simulink model "Model_plane9Old_vers"  (R2021a)
settings: Solver=FixedStepAuto  StartTime=0  StopTime=3000  FixedStep=0.1  RelTol=1e-3
model workspace (MAT data in the model file):
  Alfa = [-2 4 10 16]
  Alfa_RUD = 0.7
  Alfa_table = [-4 0 5 10 20]
  Alfa_y = [-4 6 8 9 10 12 14]
  Cxa_table = [0.03434  0.0358  0.04274; 0.02598  0.0252  0.0262; 0.04151  0.0505  0.0883; 0.122  0.1649  0.2341; 0.502  0.538  0.666]
  Cy_DB = [0.01242 0.01286 0.01457]
  Cy_fi = [0.00623 0.00643 0.00626]
  Cya = [-0.276  -0.33  -0.39; 0.859  0.991  0.82; 1.085  1.211  1.1; 1.2  1.275  1.031; 1.296  1.29  1.018; 1.45  1.178  1.043; 1.461  1.163  1.081]
  Del_B = -5
  H = [339 3256 4060 8000 12000]
  H0 = 5000
  H_table = [0 2000 4000 6000 8000 10000]
  L0 = 0
  M_C = [0.4 0.6 0.82]
  M_mz = [0.2 0.4 0.6 0.8]
  M_mz2 = [0.4 0.7 0.85]
  M_table = [0.4 0.7 0.82]
  M_y = [0.4 0.7 0.82]
  P = [50000 40000 32000 25600 20480]
  Skr = 131
  Vx0 = 160
  Vy0 = 0
  a_table = [340.3 339.5 338.8 338 337.2 336.4]
  ba = 3.466
  fi = 0
  fi_P = 2
  g = 9.81
  lz = 4500000
  mla = 60000
  mz_DB = [-0.035 -0.0358 -0.037 -0.0377]
  mz_alfa = [-0.0282 -0.0282 -0.0289 -0.0404]
  mz_alfa2 = [-8.163  -8.762  -9.714; -8.163  -8.762  -9.583; -7.975  -7.991  -7.868; -6.514  -6.413  -6.732]
  mz_fi = [-0.0695 -0.0714 -0.0739 -0.0832]
  mz_omz = [-23.768  -25.3  -28.284; -23.768  -25.3  -27.903; -23.222  -22.6  -23.32; -18.967  -18.52  -19.601]
  n_dvig = 2
  out = Simulink.SimulationOutput
  out.Data.tout = [0 1.67688873362e-06 9.33181354111e-06 4.76064375786e-05 0.000238979557766 0.0011958451587 0.00598017316339 0.0291858115735 0.107609227908 0.294605508218 0.534390352194 0.619831316604 ... (6422 elements, 6422x1)]
  out.Metadata = Simulink.SimulationMetadata
  out.Metadata.ModelInfo.ModelName = 'Model_plane2'
  out.Metadata.ModelInfo.ModelVersion = '1.11'
  out.Metadata.ModelInfo.ModelFilePath = 'C:\Users\Анастасия\Универ\Mathlab\Модель самолёта\Model_plane2.slx'
  out.Metadata.ModelInfo.UserID = 'Анастасия'
  out.Metadata.ModelInfo.MachineName = 'DESKTOP-OE36224'
  out.Metadata.ModelInfo.Platform = 'PCWIN64'
  out.Metadata.ModelInfo.ModelStructuralChecksum = [329193822; 1830100004; 2373400892; 4162968501]
  out.Metadata.ModelInfo.SimulationMode = 'normal'
  out.Metadata.ModelInfo.StartTime = 0
  out.Metadata.ModelInfo.StopTime = 100
  out.Metadata.ModelInfo.SolverInfo.Type = 'Variable-Step'
  out.Metadata.ModelInfo.SolverInfo.Solver = 'ode45'
  out.Metadata.ModelInfo.SolverInfo.MaxStepSize = 2
  out.Metadata.ModelInfo.SimulinkVersion.Name = 'Simulink'
  out.Metadata.ModelInfo.SimulinkVersion.Version = '24.1'
  out.Metadata.ModelInfo.SimulinkVersion.Release = '(R2024a)'
  out.Metadata.ModelInfo.SimulinkVersion.Date = '19-Nov-2023'
  out.Metadata.ModelInfo.LoggingInfo.LoggingToFile = 'off'
  out.Metadata.TimingInfo.WallClockTimestampStart = '2025-02-14 11:01:22'
  out.Metadata.TimingInfo.WallClockTimestampStop = '2025-02-14 11:01:24'
  out.Metadata.TimingInfo.InitializationElapsedWallTime = 1.1990057
  out.Metadata.TimingInfo.ExecutionElapsedWallTime = 1.0786509
  out.Metadata.TimingInfo.TerminationElapsedWallTime = 0.0112241
  out.Metadata.TimingInfo.TotalElapsedWallTime = 2.2888807
  out.Metadata.TimingInfo.ProfilerData = 'Profiler is not enabled'
  out.Metadata.ExecutionInfo.StopEvent = 'ReachedStopTime'
  out.Metadata.ExecutionInfo.StopEventSource = []
  out.Metadata.ExecutionInfo.StopEventDescription = 'Reached stop time of 100'
  out.Metadata.ExecutionInfo.ErrorDiagnostic = []
  out.Metadata.ExecutionInfo.WarningDiagnostics.Diagnostic = MSLDiagnostic
  out.Metadata.ExecutionInfo.WarningDiagnostics.Diagnostic.identifier = 'Simulink:blocks:DivideByZero'
  out.Metadata.ExecutionInfo.WarningDiagnostics.Diagnostic.message = 'Division by zero in ''<a href="matlab:open_and_hilite_hyperlink (''Model_plane2/Уравнения продольного движения в связанной системе координат/Блок расчёта угла атаки Alfa/Divide'',''error'')">Model_plane2/Уравнения продольного движения в связанной системе координат/Блок расчёта угла атаки Alfa/Divide</a>'''
  out.Metadata.ExecutionInfo.WarningDiagnostics.Diagnostic.paths = {'Model_plane2/Уравнения продольного движения в связанной системе координат/Блок расчёта угла атаки Alfa/Divide'}
  out.Metadata.ExecutionInfo.WarningDiagnostics.Diagnostic.arguments = {'Model_plane2/Уравнения продольного движения в связанной системе координат/Блок расчёта угла атаки Alfa/Divide'}
  out.Metadata.ExecutionInfo.WarningDiagnostics.Diagnostic.stack = struct([])
  out.Metadata.ExecutionInfo.WarningDiagnostics.Diagnostic.actionProp = '22 serialization::archive 19 0 0 0  0 1 0 0 1 1 0 0 0 0 0 1 47 SL_SERVICES:utils:EMBEDDED____ACTION____WRAPPER 2 2 0 0 183 0 109 97 116 108 97 98 58 83 105 109 117 108 105 110 107 46 83 117 112 112 114 101 115 115 101 100 68 105 97 103 110 111 115 116 105 99 40 123 39 77 111 100 101 108 95 112 108 97 110 101 50 47 1059 1088 1072 1074 1085 1077 1085 1080 1103 32 1087 1088 1086 1076 1086 1083 1100 1085 1086 1075 1086 32 1076 1074 1080 1078 1077 1085 1080 1103 32 1074 32 1089 1074 1103 1079 1072 1085 1085 1086 1081 32 1089 1080 1089 1090 1077 1084 1077 32 1082 1086 1086 1088 1076 1080 1085 1072 1090 47 1041 1083 1086 1082 32 1088 1072 1089 1095 1105 1090 1072 32 1091 1075 1083 1072 32 1072 1090 1072 1082 1080 32 65 108 102 97 47 68 105 118 105 100 101 39 125 44 39 83 105 109 117 108 105 110 107 58 98 108 111 99 107 115 58 68 105 118 105 100 101 66 121 90 101 114 111 39 41 59 2 0 0 1 6 0 0 0 0 0  1 0 0 0 0'
  out.Metadata.ExecutionInfo.WarningDiagnostics.Diagnostic.metaDataProp.UI = []
  out.Metadata.ExecutionInfo.WarningDiagnostics.Diagnostic.metaDataProp.STAGE = []
  out.Metadata.ExecutionInfo.WarningDiagnostics.Diagnostic.metaDataProp.CATEGORY = []
  out.Metadata.ExecutionInfo.WarningDiagnostics.Diagnostic.metaDataProp.COMPONENT = []
  out.Metadata.ExecutionInfo.WarningDiagnostics.Diagnostic.metaDataProp.MDL_NAME = []
  out.Metadata.ExecutionInfo.WarningDiagnostics.Diagnostic.metaDataProp.ACTION = '22 serialization::archive 19 0 0 0  0 1 0 0 1 1 0 0 0 0 0 1 47 SL_SERVICES:utils:EMBEDDED____ACTION____WRAPPER 2 2 0 0 183 0 109 97 116 108 97 98 58 83 105 109 117 108 105 110 107 46 83 117 112 112 114 101 115 115 101 100 68 105 97 103 110 111 115 116 105 99 40 123 39 77 111 100 101 108 95 112 108 97 110 101 50 47 1059 1088 1072 1074 1085 1077 1085 1080 1103 32 1087 1088 1086 1076 1086 1083 1100 1085 1086 1075 1086 32 1076 1074 1080 1078 1077 1085 1080 1103 32 1074 32 1089 1074 1103 1079 1072 1085 1085 1086 1081 32 1089 1080 1089 1090 1077 1084 1077 32 1082 1086 1086 1088 1076 1080 1085 1072 1090 47 1041 1083 1086 1082 32 1088 1072 1089 1095 1105 1090 1072 32 1091 1075 1083 1072 32 1072 1090 1072 1082 1080 32 65 108 102 97 47 68 105 118 105 100 101 39 125 44 39 83 105 109 117 108 105 110 107 58 98 108 111 99 107 115 58 68 105 118 105 100 101 66 121 90 101 114 111 39 41 59 2 0 0 1 6 0 0 0 0 0  1 0 0 0 0'
  out.Metadata.ExecutionInfo.WarningDiagnostics.Diagnostic.metaDataProp.DOC = []
  out.Metadata.ExecutionInfo.WarningDiagnostics.Diagnostic.metaDataProp.SUB_CATEGORY = []
  out.Metadata.ExecutionInfo.WarningDiagnostics.Diagnostic.metaDataProp.MSTACK_PRESERVE = []
  out.Metadata.ExecutionInfo.WarningDiagnostics.Diagnostic.metaDataProp.DOUBLE_ARGS = []
  out.Metadata.ExecutionInfo.WarningDiagnostics.Diagnostic.metaDataProp.USER_DATA = []
  out.Metadata.ExecutionInfo.WarningDiagnostics.Diagnostic.priority = 2
  out.Metadata.ExecutionInfo.WarningDiagnostics.SimulationPhase = 'Execution'
  out.Metadata.ExecutionInfo.WarningDiagnostics.SimulationTime = 0
  out.Metadata.AppInfo = struct()
  pitch0 = 0
  q_table = [1.225 1.0065 0.8194 0.6601 0.5258 0.4135]
  wz0 = 0
  xy = [24000 6200]
libraries: simulink x1
settings Model: Creator=Анастасия  LastModifiedBy=Анастасия
settings SolverCC: MaxConsecutiveMinStep=5
settings DebuggingCC: UnconnectedInputMsg=none  UnconnectedOutputMsg=none  UnconnectedLineMsg=none
settings ModelReferenceCC: EnableRefExpFcnMdlSchedulingChecks=off
settings RTWCC: Description=Generic Real-Time Target  GPUComputeCapability=5.0  DLArmComputeVersion=20.02.1

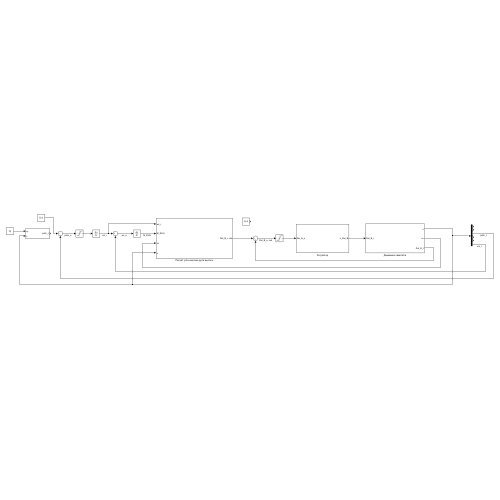
[thumbnail: Simulink's stored preview of the top-level diagram]
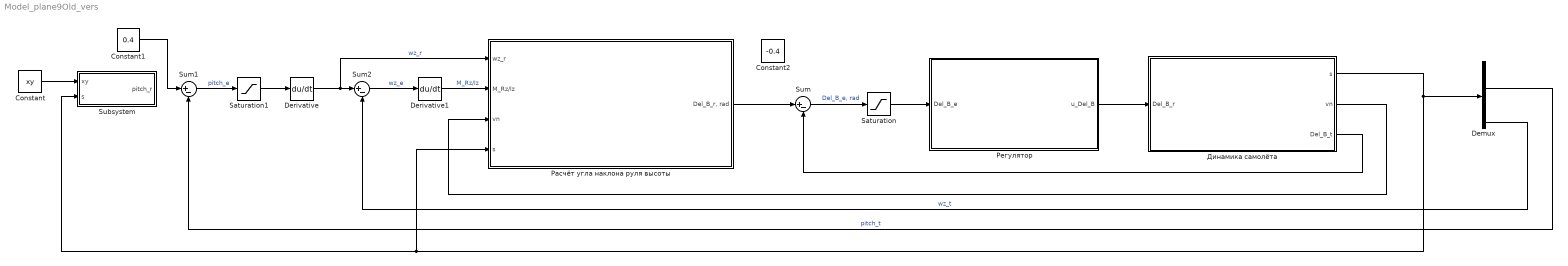
== system Model_plane9Old_vers ==
  Constant : Constant  Value=xy
  Constant1 : Constant  Value=0.4
  Constant2 : Constant  Value=-0.4
  Demux : Demux  Outputs=6
  Derivative : Derivative
  Derivative1 : Derivative
  Saturation : Saturate  UpperLimit=+0.44  LowerLimit=-0.52
  Saturation1 : Saturate  UpperLimit=+80  LowerLimit=-80
  Subsystem : Subsystem
  Sum : Sum  Inputs=|+-
  Sum1 : Sum  Inputs=|+-
  Sum2 : Sum  Inputs=|+-
  Динамика самолёта : Subsystem
  Расчёт угла наклона руля высоты : Subsystem
  Регулятор : Subsystem
  wires:
  Регулятор/1(u_Del_B) -> Динамика самолёта/1(Del_B_r)
  Sum/1 -> Saturation/1  "Del_B_e, rad"
  Динамика самолёта/1(s) -> Subsystem/2(s), Расчёт угла наклона руля высоты/4(s), Demux/1
  Constant/1 -> Subsystem/1(xy)
  Demux/3 -> Sum1/2  "pitch_t"
  Sum1/1 -> Saturation1/1  "pitch_e"
  Saturation1/1 -> Derivative/1
  Derivative/1 -> Расчёт угла наклона руля высоты/1(wz_r), Sum2/1  "wz_r"
  Demux/6 -> Sum2/2  "wz_t"
  Sum2/1 -> Derivative1/1  "wz_e"
  Derivative1/1 -> Расчёт угла наклона руля высоты/2(M_Rz/lz)  "M_Rz/lz"
  Динамика самолёта/2(vn) -> Расчёт угла наклона руля высоты/3(vn)
  Saturation/1 -> Регулятор/1(Del_B_e)
  Динамика самолёта/3(Del_B_t) -> Sum/2
  Расчёт угла наклона руля высоты/1("Del_B_r, rad") -> Sum/1
  Constant1/1 -> Sum1/1

== system Model_plane9Old_vers/Subsystem ==
  xy : Inport
  s : Inport  Port=2
  MATLAB Function : MATLAB Function  TreatAsAtomicUnit=on
  pitch_r : Outport
  wires:
  xy/1 -> MATLAB Function/1(xy)
  s/1 -> MATLAB Function/2(s)
  MATLAB Function/1(pitch) -> pitch_r/1

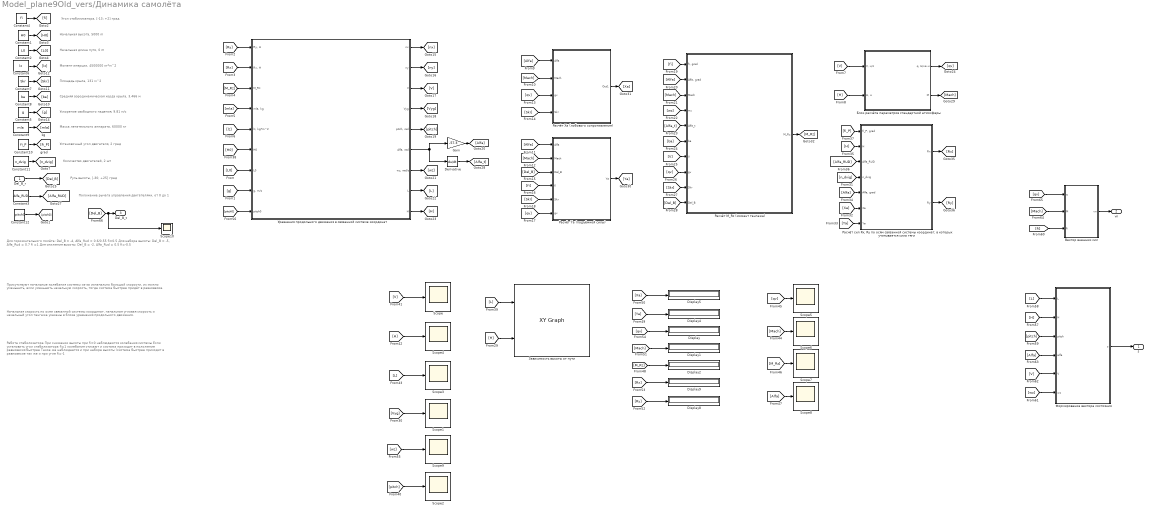
== system Model_plane9Old_vers/Динамика самолёта ==
  note: Руль высоты, [-30; +25] град
  note: Начальная скорость по осям связанной системы координат, начальная угловая скорость и начальный угол тангажа указаны в блоке уравнения продольного движения.
  note: Количество двигателей, 2 шт
  note: Присутствуют начальные колебания системы из-за изначально большой скорости, их можно уменьшить, если уменьшить начальную скорость, тогда система быстрее придёт в равновесие.
  note: Установочный угол двигателя, 2 град
  note: Ускорение свободного падения, 9.81 м/c
  note: Масса летательного аппарата, 60000 кг
  note: Положение рычага управления двигателями, от 0 до 1
  note: Для горизонтального полёта:
      | Del_B = -4, Alfa_Rud = 0.6/0.55 fi=0.5
      | Для набора высоты:
      | Del_B = -5, Alfa_Rud = 0.7 fi =1
      | Для снижения высоты:
      | Del_B = -2, Alfa_Rud = 0.5 fi=-0.5
  note: Начальная длина пути, 0 m
  note: Работа стабилизатора
      | При снижении высоты при fi=0 наблюдаются колебания системы
      | Если установить угол стабилизатора fi=1 колебания стихают и систама приходит в положение равновесия быстрее
      | Такое же наблюдается и при наборе высоты (система быстрее приходит в равновесие так же и при угле fi=-1
  note: Средняя аэродинамическая хорда крыла, 3.466 м
  note: Площадь крыла, 131 м^2
  note: Начальная высота, 5000 m
  note: Момент инерции, 4500000 кг*м^2
  note: Угол стабилизатора, [-13; +2] град
  Del_B_r : Inport
  Constant1 : Constant  Value=H0
  Constant10 : Constant  Value=fi_P
  Constant11 : Constant  Value=n_dvig
  Constant12 : Constant  Value=pitch0
  Constant2 : Constant  Value=L0
  Constant3 : Constant  Value=Alfa_RUD
  Constant4 : Constant  Value=fi
  Constant5 : Constant  Value=g
  Constant6 : Constant  Value=lz
  Constant7 : Constant  Value=Skr
  Constant8 : Constant  Value=ba
  Constant9 : Constant  Value=mla
  Derivative : Derivative
  Display{,1..2,4..5,8..9} (7 alike) : Display
  Gain : Gain  Gain=-57.3
  Scope{,1..10} (11 alike) : Scope
  Блок расчёта параметров стандартной атмосферы : Subsystem
  Вектор внешних сил : Subsystem
  Зависимость высоты от пути : simulink/Sinks/XY Graph  xmin=-1  xmax=1  ymin=-1  ymax=1  st=-1
  Расчёт M_Rz (момент тангажа) : Subsystem
  Расчёт Xa (лобового сопротивления) : Subsystem
  Расчёт Ya (подъёмной силы) : Subsystem
  "Расчёт сил Rx, Ry по осям связанной системы координат, в которых учитывается сила тяги" : Subsystem
  Уравнения продольного движения в связанной системе координат : Subsystem
  Формирование вектора состояния : Subsystem
  s : Outport
  vn : Outport  Port=2
  Del_B_t : Outport  Port=3
  wires:
  [pitch0] -> Уравнения продольного движения в связанной системе координат/9(pitch0)
  Constant12/1 -> [pitch0]
  [wz] -> Scope9/1
  Constant1/1 -> [H0]
  Уравнения продольного движения в связанной системе координат/9(H) -> [H]
  Блок расчёта параметров стандартной атмосферы/1("q, Н/кв.м") -> [qv]
  [M_Rz] -> Display2/1
  [qv] -> Расчёт Ya (подъёмной силы)/6(gv)
  Gain/1 -> [Alfa]
  Расчёт M_Rz (момент тангажа)/1(M_Rz) -> [M_Rz]
  [L0] -> Уравнения продольного движения в связанной системе координат/7(L0)
  [H0] -> Уравнения продольного движения в связанной системе координат/6(H0)
  [qv] -> Display/1
  [Rx] -> Display9/1
  [lz] -> Уравнения продольного движения в связанной системе координат/5("lz, kg*m^2")
  Constant5/1 -> [g]
  [qv] -> Расчёт Xa (лобового сопротивления)/3(gv)
  [pitch] -> Scope2/1
  [Ry] -> Display8/1
  [Vyg] -> Scope1/1
  [Xa] -> Display5/1
  Уравнения продольного движения в связанной системе координат/1(nx) -> [nx]
  Derivative/1 -> [Alfa_t]
  [Mach] -> Display1/1
  [Xa] -> "Расчёт сил Rx, Ry по осям связанной системы координат, в которых учитывается сила тяги"/6(Xa)
  [ba] -> Расчёт M_Rz (момент тангажа)/6(ba)
  [M_Rz] -> Scope7/1
  [Mach] -> Scope6/1
  Constant9/1 -> [mla]
  [H] -> Блок расчёта параметров стандартной атмосферы/2("H, м")
  [Ya] -> Display4/1
  [fi] -> Расчёт M_Rz (момент тангажа)/1("fi, grad")
  [fi_P] -> "Расчёт сил Rx, Ry по осям связанной системы координат, в которых учитывается сила тяги"/1("fi_P, grad")
  [L] -> Scope3/1
  [L] -> Зависимость высоты от пути/1
  [H] -> Scope4/1
  [V] -> Scope/1
  [Ya] -> "Расчёт сил Rx, Ry по осям связанной системы координат, в которых учитывается сила тяги"/7(Ya)
  [V] -> Расчёт M_Rz (момент тангажа)/7(V)
  [Alfa] -> Расчёт M_Rz (момент тангажа)/2("Alfa, grad")
  Уравнения продольного движения в связанной системе координат/5("pitch, rad") -> [pitch]
  [Del_B] -> Расчёт Ya (подъёмной силы)/3(Del_B)
  [Skr] -> Расчёт M_Rz (момент тангажа)/9(Skr)
  [Alfa_RUD] -> "Расчёт сил Rx, Ry по осям связанной системы координат, в которых учитывается сила тяги"/3(Alfa_RUD)
  "Расчёт сил Rx, Ry по осям связанной системы координат, в которых учитывается сила тяги"/1(Rx) -> [Rx]
  [H] -> "Расчёт сил Rx, Ry по осям связанной системы координат, в которых учитывается сила тяги"/2(H)
  [H] -> Зависимость высоты от пути/2
  [fi] -> Расчёт Ya (подъёмной силы)/4(fi)
  Расчёт Xa (лобового сопротивления)/1(Out1) -> [Xa]
  [Del_B] -> Расчёт M_Rz (момент тангажа)/10(Del_B)
  [n_dvig] -> "Расчёт сил Rx, Ry по осям связанной системы координат, в которых учитывается сила тяги"/4(n_dvig)
  [Alfa_t] -> Расчёт M_Rz (момент тангажа)/5(Alfa_t)
  [wz] -> Расчёт M_Rz (момент тангажа)/4(wz)
  Блок расчёта параметров стандартной атмосферы/2(М) -> [Mach]
  Уравнения продольного движения в связанной системе координат/7("wz, rad/s") -> [wz]
  [qv] -> Scope5/1
  [Rx] -> Уравнения продольного движения в связанной системе координат/2("Rx, H")
  Уравнения продольного движения в связанной системе координат/6("Alfa, rad") -> Derivative/1, Gain/1
  "Расчёт сил Rx, Ry по осям связанной системы координат, в которых учитывается сила тяги"/2(Ry) -> [Ry]
  [qv] -> Расчёт M_Rz (момент тангажа)/8(gv)
  [Mach] -> Расчёт Xa (лобового сопротивления)/2(Mach)
  [mla] -> Уравнения продольного движения в связанной системе координат/4("mla, kg")
  [Mach] -> Расчёт Ya (подъёмной силы)/2(Mach)
  Уравнения продольного движения в связанной системе координат/8(L) -> [L]
  [Alfa] -> "Расчёт сил Rx, Ry по осям связанной системы координат, в которых учитывается сила тяги"/5("Alfa, grad")
  [Skr] -> Расчёт Ya (подъёмной силы)/5(Skr)
  [Alfa] -> Расчёт Xa (лобового сопротивления)/1(Alfa)
  Constant10/1 -> [fi_P]
  Constant3/1 -> [Alfa_RUD]
  [M_Rz] -> Уравнения продольного движения в связанной системе координат/3(M_Rz)
  [Mach] -> Расчёт M_Rz (момент тангажа)/3(Mach)
  [V] -> Блок расчёта параметров стандартной атмосферы/1("V, м/с")
  [g] -> Уравнения продольного движения в связанной системе координат/8("g, m/s")
  Уравнения продольного движения в связанной системе координат/2(ny) -> [ny]
  [Alfa] -> Scope8/1
  Уравнения продольного движения в связанной системе координат/4(Vyg) -> [Vyg]
  Расчёт Ya (подъёмной силы)/1(Ya) -> [Ya]
  Уравнения продольного движения в связанной системе координат/3(V) -> [V]
  [Alfa] -> Расчёт Ya (подъёмной силы)/1(Alfa)
  Constant6/1 -> [lz]
  Constant8/1 -> [ba]
  Constant2/1 -> [L0]
  [Ry] -> Уравнения продольного движения в связанной системе координат/1("Ry, H")
  Constant7/1 -> [Skr]
  Constant11/1 -> [n_dvig]
  [Skr] -> Расчёт Xa (лобового сопротивления)/4(Skr)
  Формирование вектора состояния/1(s) -> s/1
  [pitch] -> Формирование вектора состояния/3(pitch)
  [V] -> Формирование вектора состояния/5(V)
  [Alfa] -> Формирование вектора состояния/4(alfa)
  Вектор внешних сил/1(vn) -> vn/1
  [qv] -> Вектор внешних сил/1(q)
  [Mach] -> Вектор внешних сил/2(M)
  Constant4/1 -> [fi]
  [H] -> Формирование вектора состояния/2(H)
  [L] -> Формирование вектора состояния/1(L)
  Del_B_r/1 -> [Del_B]
  [wz] -> Формирование вектора состояния/6(wz)
  [fi] -> Вектор внешних сил/3(fi)
  [Del_B] -> Scope10/1, Del_B_t/1

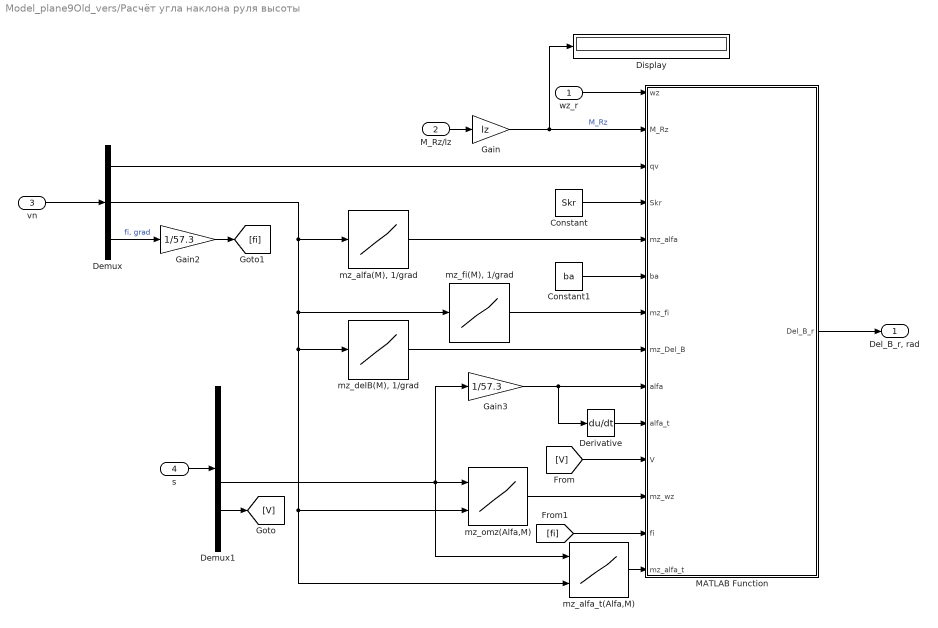
== system Model_plane9Old_vers/Расчёт угла наклона руля высоты ==
  wz_r : Inport
  M_Rz/lz : Inport  Port=2
  vn : Inport  Port=3
  s : Inport  Port=4
  Constant : Constant  Value=Skr
  Constant1 : Constant  Value=ba
  Demux : Demux  Outputs=3
  Demux1 : Demux  Outputs=6
  Derivative : Derivative
  Display : Display
  Gain : Gain  Gain=lz
  Gain2 : Gain  Gain=1/57.3
  Gain3 : Gain  Gain=1/57.3
  MATLAB Function : MATLAB Function  TreatAsAtomicUnit=on
  "mz_alfa(M), 1/grad" : Lookup_n-D  NumberOfTableDimensions=1  BreakpointsForDimension1=M_mz  Table=mz_alfa  InternalRulePriority=Speed  RndMeth=Simplest  InputSameDT=on
  mz_alfa_t(Alfa,M) : Lookup_n-D  BreakpointsForDimension1=Alfa  BreakpointsForDimension2=M_mz2  Table=mz_alfa2  InternalRulePriority=Speed  RndMeth=Simplest  InputSameDT=on
      settings: InputPortMap=u0,u1
  "mz_delB(M), 1/grad" : Lookup_n-D  NumberOfTableDimensions=1  BreakpointsForDimension1=M_mz  Table=mz_DB  InternalRulePriority=Speed  RndMeth=Simplest  InputSameDT=on
  "mz_fi(M), 1/grad" : Lookup_n-D  NumberOfTableDimensions=1  BreakpointsForDimension1=M_mz  Table=mz_fi  InternalRulePriority=Speed  RndMeth=Simplest  InputSameDT=on
  mz_omz(Alfa,M) : Lookup_n-D  BreakpointsForDimension1=Alfa  BreakpointsForDimension2=M_mz2  Table=mz_omz  InternalRulePriority=Speed  RndMeth=Simplest  InputSameDT=on
      settings: InputPortMap=u0,u1
  "Del_B_r, rad" : Outport
  wires:
  M_Rz/lz/1 -> Gain/1
  Gain/1 -> Display/1, MATLAB Function/2(M_Rz)  "M_Rz"
  wz_r/1 -> MATLAB Function/1(wz)
  MATLAB Function/1(Del_B_r) -> "Del_B_r, rad"/1
  vn/1 -> Demux/1
  Demux/1 -> MATLAB Function/3(qv)
  Demux1/4 -> mz_alfa_t(Alfa,M)/1, mz_omz(Alfa,M)/1, Gain3/1
  Demux/2 -> mz_alfa_t(Alfa,M)/2, mz_omz(Alfa,M)/2, "mz_delB(M), 1/grad"/1, "mz_fi(M), 1/grad"/1, "mz_alfa(M), 1/grad"/1
  Demux/3 -> Gain2/1  "fi, grad"
  s/1 -> Demux1/1
  Gain3/1 -> Derivative/1, MATLAB Function/9(alfa)
  Constant/1 -> MATLAB Function/4(Skr)
  "mz_alfa(M), 1/grad"/1 -> MATLAB Function/5(mz_alfa)
  Constant1/1 -> MATLAB Function/6(ba)
  "mz_fi(M), 1/grad"/1 -> MATLAB Function/7(mz_fi)
  "mz_delB(M), 1/grad"/1 -> MATLAB Function/8(mz_Del_B)
  mz_alfa_t(Alfa,M)/1 -> MATLAB Function/14(mz_alfa_t)
  mz_omz(Alfa,M)/1 -> MATLAB Function/12(mz_wz)
  Derivative/1 -> MATLAB Function/10(alfa_t)
  Demux1/5 -> [V]
  [V] -> MATLAB Function/11(V)
  Gain2/1 -> [fi]
  [fi] -> MATLAB Function/13(fi)

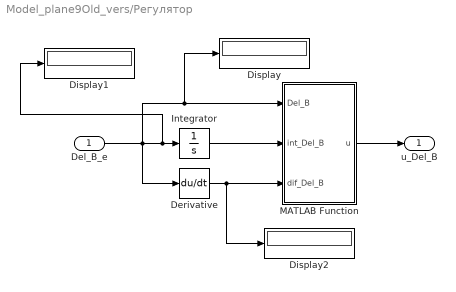
== system Model_plane9Old_vers/Регулятор ==
  Del_B_e : Inport
  Derivative : Derivative
  Display : Display
  Display1 : Display
  Display2 : Display
  Integrator : Integrator
  MATLAB Function : MATLAB Function  TreatAsAtomicUnit=on
  u_Del_B : Outport
  wires:
  Del_B_e/1 -> Derivative/1, Display/1, MATLAB Function/1(Del_B), Display1/1, Integrator/1
  MATLAB Function/1(u) -> u_Del_B/1
  Integrator/1 -> MATLAB Function/2(int_Del_B)
  Derivative/1 -> Display2/1, MATLAB Function/3(dif_Del_B)

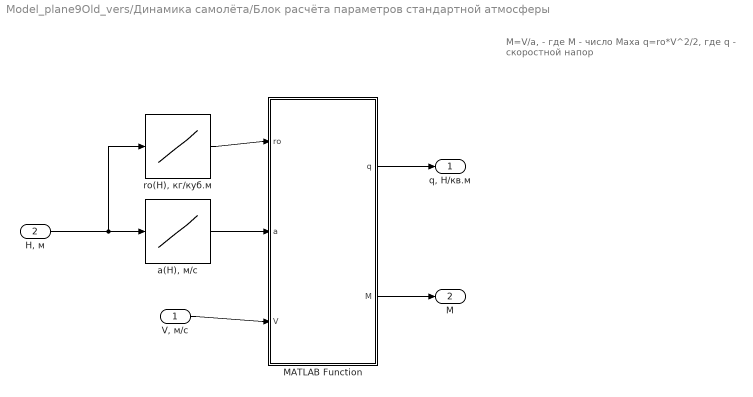
== system Model_plane9Old_vers/Динамика самолёта/Блок расчёта параметров стандартной атмосферы ==
  note: M=V/a, - где М - число Маха
      | q=ro*V^2/2, где q - скоростной напор
  "V, м/с" : Inport
  "H, м" : Inport  Port=2
  MATLAB Function : MATLAB Function  TreatAsAtomicUnit=on
  "a(H), м/с" : Lookup_n-D  NumberOfTableDimensions=1  BreakpointsForDimension1=H_table  Table=a_table  InternalRulePriority=Speed  RndMeth=Simplest  InputSameDT=on
  "ro(H), кг/куб.м" : Lookup_n-D  NumberOfTableDimensions=1  BreakpointsForDimension1=H_table  Table=q_table  InternalRulePriority=Speed  RndMeth=Simplest  InputSameDT=on
  "q, Н/кв.м" : Outport
  М : Outport  Port=2
  wires:
  "H, м"/1 -> "ro(H), кг/куб.м"/1, "a(H), м/с"/1
  "ro(H), кг/куб.м"/1 -> MATLAB Function/1(ro)
  "a(H), м/с"/1 -> MATLAB Function/2(a)
  MATLAB Function/1(q) -> "q, Н/кв.м"/1
  MATLAB Function/2(M) -> М/1
  "V, м/с"/1 -> MATLAB Function/3(V)

== system Model_plane9Old_vers/Динамика самолёта/Вектор внешних сил ==
  q : Inport
  M : Inport  Port=2
  fi : Inport  Port=3
  MATLAB Function : MATLAB Function  TreatAsAtomicUnit=on
  vn : Outport
  wires:
  M/1 -> MATLAB Function/2(M)
  q/1 -> MATLAB Function/1(q)
  MATLAB Function/1(vn) -> vn/1
  fi/1 -> MATLAB Function/3(fi)

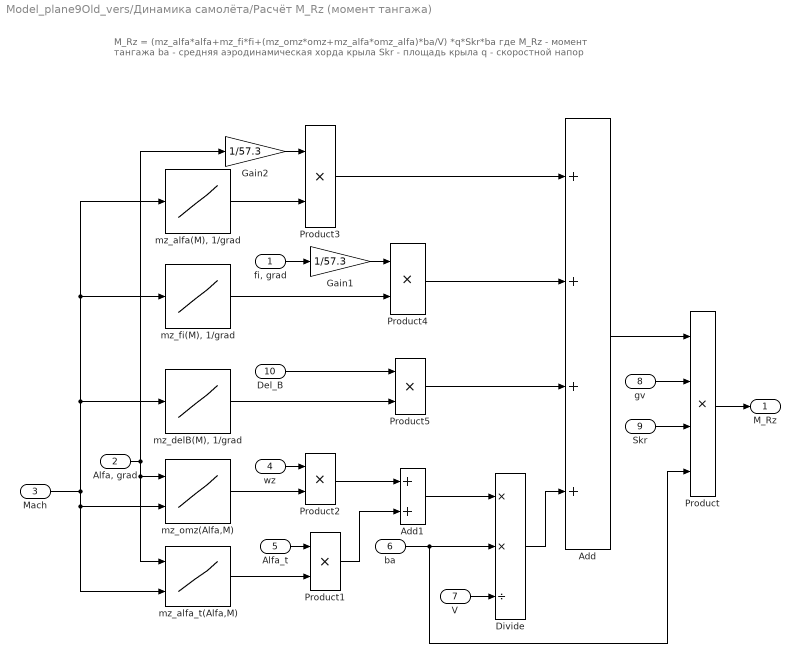
== system Model_plane9Old_vers/Динамика самолёта/Расчёт M_Rz (момент тангажа) ==
  note: M_Rz = (mz_alfa*alfa+mz_fi*fi+(mz_omz*omz+mz_alfa*omz_alfa)*ba/V) *q*Skr*ba
      | где M_Rz - момент тангажа
      | ba - средняя аэродинамическая хорда крыла
      | Skr - площадь крыла
      | q - скоростной напор
  "fi, grad" : Inport
  "Alfa, grad" : Inport  Port=2
  Mach : Inport  Port=3
  wz : Inport  Port=4
  Alfa_t : Inport  Port=5
  ba : Inport  Port=6
  V : Inport  Port=7
  gv : Inport  Port=8
  Skr : Inport  Port=9
  Del_B : Inport  Port=10
  Add : Sum  Inputs=++++
  Add1 : Sum
  Divide : Product  Inputs=**/
  Gain1 : Gain  Gain=1/57.3
  Gain2 : Gain  Gain=1/57.3
  Product : Product  Inputs=4
  Product{1..5} (5 alike) : Product
  "mz_alfa(M), 1/grad" : Lookup_n-D  NumberOfTableDimensions=1  BreakpointsForDimension1=M_mz  Table=mz_alfa  InternalRulePriority=Speed  RndMeth=Simplest  InputSameDT=on
  mz_alfa_t(Alfa,M) : Lookup_n-D  BreakpointsForDimension1=Alfa  BreakpointsForDimension2=M_mz2  Table=mz_alfa2  InternalRulePriority=Speed  RndMeth=Simplest  InputSameDT=on
      settings: InputPortMap=u0,u1
  "mz_delB(M), 1/grad" : Lookup_n-D  NumberOfTableDimensions=1  BreakpointsForDimension1=M_mz  Table=mz_DB  InternalRulePriority=Speed  RndMeth=Simplest  InputSameDT=on
  "mz_fi(M), 1/grad" : Lookup_n-D  NumberOfTableDimensions=1  BreakpointsForDimension1=M_mz  Table=mz_fi  InternalRulePriority=Speed  RndMeth=Simplest  InputSameDT=on
  mz_omz(Alfa,M) : Lookup_n-D  BreakpointsForDimension1=Alfa  BreakpointsForDimension2=M_mz2  Table=mz_omz  InternalRulePriority=Speed  RndMeth=Simplest  InputSameDT=on
      settings: InputPortMap=u0,u1
  M_Rz : Outport
  wires:
  Product/1 -> M_Rz/1
  ba/1 -> Product/4, Divide/2
  Skr/1 -> Product/3
  gv/1 -> Product/2
  Add/1 -> Product/1
  V/1 -> Divide/3
  Divide/1 -> Add/4
  Add1/1 -> Divide/1
  Product2/1 -> Add1/1
  Product1/1 -> Add1/2
  Alfa_t/1 -> Product1/1
  wz/1 -> Product2/1
  mz_omz(Alfa,M)/1 -> Product2/2
  mz_alfa_t(Alfa,M)/1 -> Product1/2
  Mach/1 -> mz_omz(Alfa,M)/2, mz_alfa_t(Alfa,M)/2, "mz_alfa(M), 1/grad"/1, "mz_fi(M), 1/grad"/1, "mz_delB(M), 1/grad"/1
  "mz_alfa(M), 1/grad"/1 -> Product3/2
  "mz_fi(M), 1/grad"/1 -> Product4/2
  "mz_delB(M), 1/grad"/1 -> Product5/2
  Product3/1 -> Add/1
  Product4/1 -> Add/2
  Product5/1 -> Add/3
  Del_B/1 -> Product5/1
  "fi, grad"/1 -> Gain1/1
  Gain1/1 -> Product4/1
  "Alfa, grad"/1 -> Gain2/1, mz_omz(Alfa,M)/1, mz_alfa_t(Alfa,M)/1
  Gain2/1 -> Product3/1

== system Model_plane9Old_vers/Динамика самолёта/Расчёт Xa (лобового сопротивления) ==
  note: Xa = Cxa*q*Skr
  Alfa : Inport
  Mach : Inport  Port=2
  gv : Inport  Port=3
  Skr : Inport  Port=4
  "Cxa(Alfa, M)" : Lookup_n-D  BreakpointsForDimension1=Alfa_table  BreakpointsForDimension2=M_table  Table=Cxa_table  InternalRulePriority=Speed  RndMeth=Simplest  InputSameDT=on
      settings: InputPortMap=u0,u1
  Product : Product  Inputs=3
  Out1 : Outport
  wires:
  Alfa/1 -> "Cxa(Alfa, M)"/1
  Product/1 -> Out1/1
  Skr/1 -> Product/3
  gv/1 -> Product/2
  Mach/1 -> "Cxa(Alfa, M)"/2
  "Cxa(Alfa, M)"/1 -> Product/1

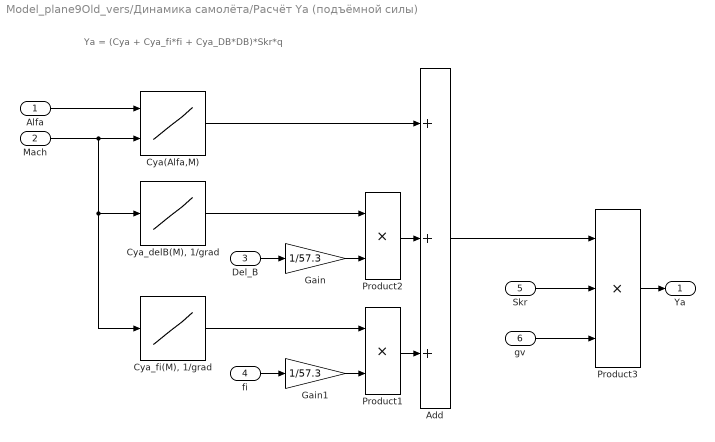
== system Model_plane9Old_vers/Динамика самолёта/Расчёт Ya (подъёмной силы) ==
  note: Ya = (Cya + Cya_fi*fi + Cya_DB*DB)*Skr*q
  Alfa : Inport
  Mach : Inport  Port=2
  Del_B : Inport  Port=3
  fi : Inport  Port=4
  Skr : Inport  Port=5
  gv : Inport  Port=6
  Add : Sum  Inputs=+++
  Cya(Alfa,M) : Lookup_n-D  BreakpointsForDimension1=Alfa_y  BreakpointsForDimension2=M_y  Table=Cya  InternalRulePriority=Speed  RndMeth=Simplest  InputSameDT=on
      settings: InputPortMap=u0,u1
  "Cya_delB(M), 1/grad" : Lookup_n-D  NumberOfTableDimensions=1  BreakpointsForDimension1=M_C  Table=Cy_DB  InternalRulePriority=Speed  RndMeth=Simplest  InputSameDT=on
  "Cya_fi(M), 1/grad" : Lookup_n-D  NumberOfTableDimensions=1  BreakpointsForDimension1=M_C  Table=Cy_fi  InternalRulePriority=Speed  RndMeth=Simplest  InputSameDT=on
  Gain : Gain  Gain=1/57.3
  Gain1 : Gain  Gain=1/57.3
  Product1 : Product
  Product2 : Product
  Product3 : Product  Inputs=3
  Ya : Outport
  wires:
  Alfa/1 -> Cya(Alfa,M)/1
  gv/1 -> Product3/3
  Skr/1 -> Product3/2
  Product3/1 -> Ya/1
  "Cya_fi(M), 1/grad"/1 -> Product1/1
  "Cya_delB(M), 1/grad"/1 -> Product2/1
  Mach/1 -> "Cya_delB(M), 1/grad"/1, "Cya_fi(M), 1/grad"/1, Cya(Alfa,M)/2
  Cya(Alfa,M)/1 -> Add/1
  Product2/1 -> Add/2
  Product1/1 -> Add/3
  Add/1 -> Product3/1
  Del_B/1 -> Gain/1
  Gain/1 -> Product2/2
  fi/1 -> Gain1/1
  Gain1/1 -> Product1/2

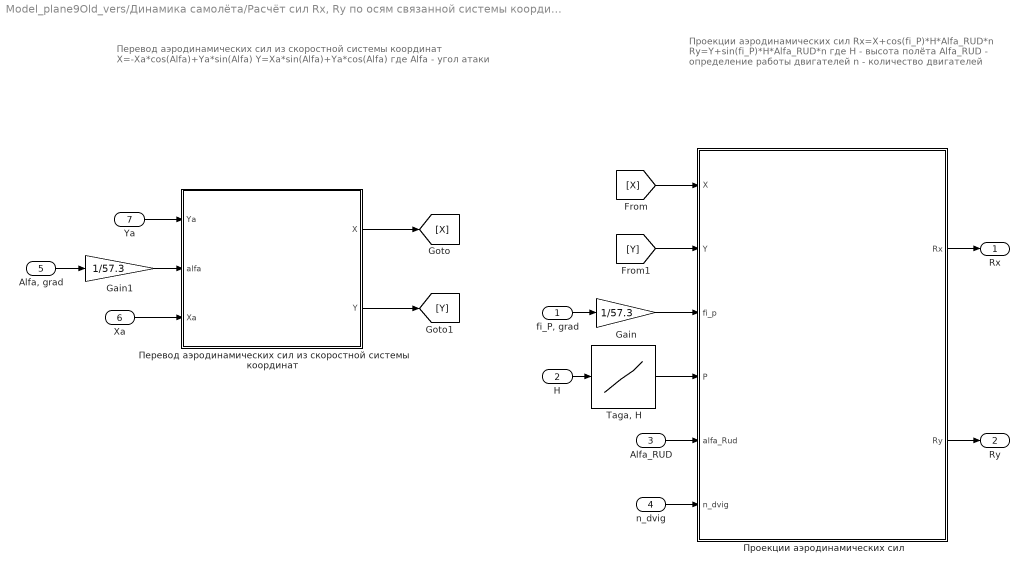
== system Model_plane9Old_vers/Динамика самолёта/Расчёт сил Rx, Ry по осям связанной системы координат, в которых учитывается сила тяги ==
  note: Проекции аэродинамических сил
      | Rx=X+cos(fi_P)*H*Alfa_RUD*n
      | Ry=Y+sin(fi_P)*H*Alfa_RUD*n
      | где Н - высота полёта
      | Alfa_RUD - определение работы двигателей
      | n - количество двигателей
  note: Перевод аэродинамических сил из скоростной системы координат
      | X=-Xa*cos(Alfa)+Ya*sin(Alfa)
      | Y=Xa*sin(Alfa)+Ya*cos(Alfa)
      | где Alfa - угол атаки
  "fi_P, grad" : Inport
  H : Inport  Port=2
  Alfa_RUD : Inport  Port=3
  n_dvig : Inport  Port=4
  "Alfa, grad" : Inport  Port=5
  Xa : Inport  Port=6
  Ya : Inport  Port=7
  Gain : Gain  Gain=1/57.3
  Gain1 : Gain  Gain=1/57.3
  "Taga, H" : Lookup_n-D  NumberOfTableDimensions=1  BreakpointsForDimension1=H  Table=P  InternalRulePriority=Speed  RndMeth=Simplest  InputSameDT=on
  Перевод аэродинамических сил из скоростной системы координат : MATLAB Function  TreatAsAtomicUnit=on
  Проекции аэродинамических сил : MATLAB Function  TreatAsAtomicUnit=on
  Rx : Outport
  Ry : Outport  Port=2
  wires:
  "fi_P, grad"/1 -> Gain/1
  H/1 -> "Taga, H"/1
  "Alfa, grad"/1 -> Gain1/1
  Перевод аэродинамических сил из скоростной системы координат/1(X) -> [X]
  Перевод аэродинамических сил из скоростной системы координат/2(Y) -> [Y]
  Ya/1 -> Перевод аэродинамических сил из скоростной системы координат/1(Ya)
  Xa/1 -> Перевод аэродинамических сил из скоростной системы координат/3(Xa)
  Gain1/1 -> Перевод аэродинамических сил из скоростной системы координат/2(alfa)
  Проекции аэродинамических сил/2(Ry) -> Ry/1
  Проекции аэродинамических сил/1(Rx) -> Rx/1
  n_dvig/1 -> Проекции аэродинамических сил/6(n_dvig)
  Alfa_RUD/1 -> Проекции аэродинамических сил/5(alfa_Rud)
  "Taga, H"/1 -> Проекции аэродинамических сил/4(P)
  Gain/1 -> Проекции аэродинамических сил/3(fi_p)
  [Y] -> Проекции аэродинамических сил/2(Y)
  [X] -> Проекции аэродинамических сил/1(X)

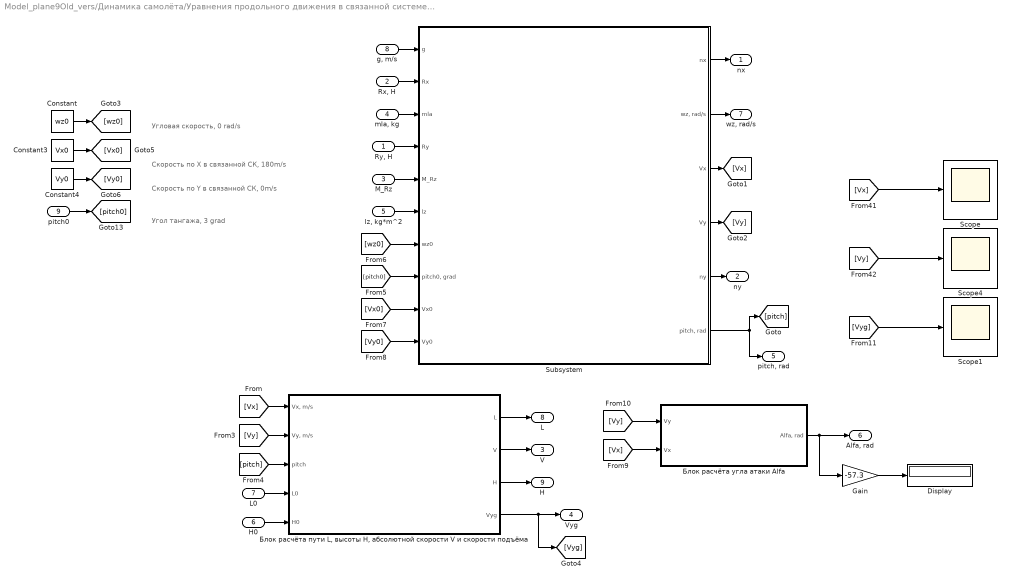
== system Model_plane9Old_vers/Динамика самолёта/Уравнения продольного движения в связанной системе координат ==
  note: Угловая скорость, 0 rad/s
  note: Скорость по X в связанной СК, 180m/s
  note: Угол тангажа, 3 grad
  note: Скорость по Y в связанной СК, 0m/s
  "Ry, H" : Inport
  "Rx, H" : Inport  Port=2
  M_Rz : Inport  Port=3
  "mla, kg" : Inport  Port=4
  "lz, kg*m^2" : Inport  Port=5
  H0 : Inport  Port=6
  L0 : Inport  Port=7
  "g, m/s" : Inport  Port=8
  pitch0 : Inport  Port=9
  Constant : Constant  Value=wz0
  Constant3 : Constant  Value=Vx0
  Constant4 : Constant  Value=Vy0
  Display : Display
  Gain : Gain  Gain=-57.3
  Scope : Scope
  Scope1 : Scope
  Scope4 : Scope
  Subsystem : Subsystem
  "Блок расчёта пути L, высоты H, абсолютной скорости V и скорости подъёма" : Subsystem
  Блок расчёта угла атаки Alfa : Subsystem
  nx : Outport
  ny : Outport  Port=2
  V : Outport  Port=3
  Vyg : Outport  Port=4
  "pitch, rad" : Outport  Port=5
  "Alfa, rad" : Outport  Port=6
  "wz, rad/s" : Outport  Port=7
  L : Outport  Port=8
  H : Outport  Port=9
  wires:
  "Блок расчёта пути L, высоты H, абсолютной скорости V и скорости подъёма"/1(L) -> L/1
  Subsystem/1(nx) -> nx/1
  Subsystem/5(ny) -> ny/1
  Subsystem/6("pitch, rad") -> "pitch, rad"/1, [pitch]
  Subsystem/3(Vx) -> [Vx]
  Subsystem/4(Vy) -> [Vy]
  Subsystem/2("wz, rad/s") -> "wz, rad/s"/1
  [Vx] -> "Блок расчёта пути L, высоты H, абсолютной скорости V и скорости подъёма"/1("Vx, m/s")
  [Vy] -> "Блок расчёта пути L, высоты H, абсолютной скорости V и скорости подъёма"/2("Vy, m/s")
  [pitch] -> "Блок расчёта пути L, высоты H, абсолютной скорости V и скорости подъёма"/3(pitch)
  L0/1 -> "Блок расчёта пути L, высоты H, абсолютной скорости V и скорости подъёма"/4(L0)
  "g, m/s"/1 -> Subsystem/1(g)
  "Rx, H"/1 -> Subsystem/2(Rx)
  "Ry, H"/1 -> Subsystem/4(Ry)
  M_Rz/1 -> Subsystem/5(M_Rz)
  "lz, kg*m^2"/1 -> Subsystem/6(lz)
  pitch0/1 -> [pitch0]
  Constant4/1 -> [Vy0]
  Constant3/1 -> [Vx0]
  Constant/1 -> [wz0]
  [pitch0] -> Subsystem/8("pitch0, grad")
  [wz0] -> Subsystem/7(wz0)
  [Vx0] -> Subsystem/9(Vx0)
  [Vy0] -> Subsystem/10(Vy0)
  "mla, kg"/1 -> Subsystem/3(mla)
  Блок расчёта угла атаки Alfa/1("Alfa, rad") -> Gain/1, "Alfa, rad"/1
  [Vy] -> Scope4/1
  [Vx] -> Scope/1
  [Vyg] -> Scope1/1
  [Vx] -> Блок расчёта угла атаки Alfa/2(Vx)
  [Vy] -> Блок расчёта угла атаки Alfa/1(Vy)
  Gain/1 -> Display/1
  "Блок расчёта пути L, высоты H, абсолютной скорости V и скорости подъёма"/2(V) -> V/1
  "Блок расчёта пути L, высоты H, абсолютной скорости V и скорости подъёма"/3(H) -> H/1
  "Блок расчёта пути L, высоты H, абсолютной скорости V и скорости подъёма"/4(Vyg) -> Vyg/1, [Vyg]
  H0/1 -> "Блок расчёта пути L, высоты H, абсолютной скорости V и скорости подъёма"/5(H0)

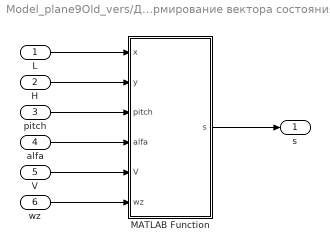
== system Model_plane9Old_vers/Динамика самолёта/Формирование вектора состояния ==
  L : Inport
  H : Inport  Port=2
  pitch : Inport  Port=3
  alfa : Inport  Port=4
  V : Inport  Port=5
  wz : Inport  Port=6
  MATLAB Function : MATLAB Function  TreatAsAtomicUnit=on
  s : Outport
  wires:
  L/1 -> MATLAB Function/1(x)
  MATLAB Function/1(s) -> s/1
  H/1 -> MATLAB Function/2(y)
  pitch/1 -> MATLAB Function/3(pitch)
  alfa/1 -> MATLAB Function/4(alfa)
  V/1 -> MATLAB Function/5(V)
  wz/1 -> MATLAB Function/6(wz)

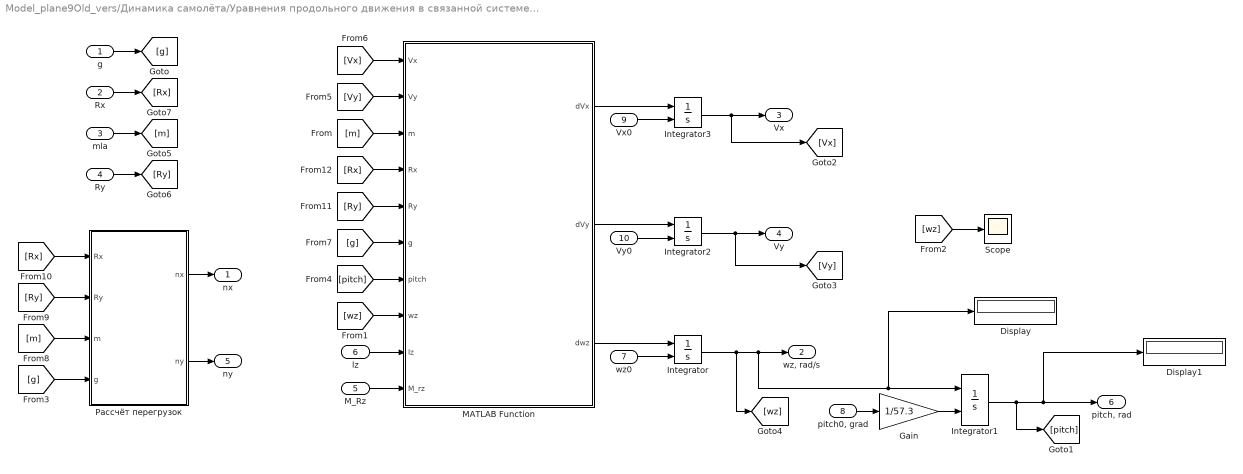
== system Model_plane9Old_vers/Динамика самолёта/Уравнения продольного движения в связанной системе координат/Subsystem ==
  g : Inport
  Rx : Inport  Port=2
  mla : Inport  Port=3
  Ry : Inport  Port=4
  M_Rz : Inport  Port=5
  lz : Inport  Port=6
  wz0 : Inport  Port=7
  "pitch0, grad" : Inport  Port=8
  Vx0 : Inport  Port=9
  Vy0 : Inport  Port=10
  Display : Display
  Display1 : Display
  Gain : Gain  Gain=1/57.3
  Integrator{,1..3} (4 alike) : Integrator  InitialConditionSource=external
  MATLAB Function : MATLAB Function  TreatAsAtomicUnit=on
  Scope : Scope
  Рассчёт перегрузок : MATLAB Function  TreatAsAtomicUnit=on
  nx : Outport
  "wz, rad/s" : Outport  Port=2
  Vx : Outport  Port=3
  Vy : Outport  Port=4
  ny : Outport  Port=5
  "pitch, rad" : Outport  Port=6
  wires:
  Vx0/1 -> Integrator3/2
  Vy0/1 -> Integrator2/2
  "pitch0, grad"/1 -> Gain/1
  Integrator2/1 -> [Vy], Vy/1
  g/1 -> [g]
  Integrator3/1 -> [Vx], Vx/1
  Gain/1 -> Integrator1/2
  wz0/1 -> Integrator/2
  Integrator1/1 -> Display1/1, "pitch, rad"/1, [pitch]
  Integrator/1 -> [wz], Integrator1/1, Display/1, "wz, rad/s"/1
  [Vy] -> MATLAB Function/2(Vy)
  [Vx] -> MATLAB Function/1(Vx)
  [g] -> MATLAB Function/6(g)
  [pitch] -> MATLAB Function/7(pitch)
  MATLAB Function/1(dVx) -> Integrator3/1
  MATLAB Function/2(dVy) -> Integrator2/1
  M_Rz/1 -> MATLAB Function/10(M_rz)
  lz/1 -> MATLAB Function/9(Iz)
  [wz] -> MATLAB Function/8(wz)
  MATLAB Function/3(dwz) -> Integrator/1
  [wz] -> Scope/1
  Рассчёт перегрузок/2(ny) -> ny/1
  Рассчёт перегрузок/1(nx) -> nx/1
  [g] -> Рассчёт перегрузок/4(g)
  mla/1 -> [m]
  [m] -> MATLAB Function/3(m)
  [m] -> Рассчёт перегрузок/3(m)
  Ry/1 -> [Ry]
  Rx/1 -> [Rx]
  [Ry] -> Рассчёт перегрузок/2(Ry)
  [Rx] -> Рассчёт перегрузок/1(Rx)
  [Ry] -> MATLAB Function/5(Ry)
  [Rx] -> MATLAB Function/4(Rx)

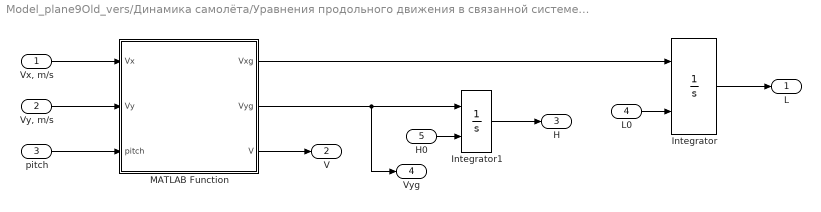
== system Model_plane9Old_vers/Динамика самолёта/Уравнения продольного движения в связанной системе координат/Блок расчёта пути L, высоты H, абсолютной скорости V и скорости подъёма ==
  "Vx, m/s" : Inport
  "Vy, m/s" : Inport  Port=2
  pitch : Inport  Port=3
  L0 : Inport  Port=4
  H0 : Inport  Port=5
  Integrator : Integrator  InitialConditionSource=external
  Integrator1 : Integrator  InitialConditionSource=external
  MATLAB Function : MATLAB Function  TreatAsAtomicUnit=on
  L : Outport
  V : Outport  Port=2
  H : Outport  Port=3
  Vyg : Outport  Port=4
  wires:
  "Vx, m/s"/1 -> MATLAB Function/1(Vx)
  "Vy, m/s"/1 -> MATLAB Function/2(Vy)
  L0/1 -> Integrator/2
  MATLAB Function/1(Vxg) -> Integrator/1
  Integrator/1 -> L/1
  pitch/1 -> MATLAB Function/3(pitch)
  H0/1 -> Integrator1/2
  Integrator1/1 -> H/1
  MATLAB Function/2(Vyg) -> Vyg/1, Integrator1/1
  MATLAB Function/3(V) -> V/1

== system Model_plane9Old_vers/Динамика самолёта/Уравнения продольного движения в связанной системе координат/Блок расчёта угла атаки Alfa ==
  Vy : Inport
  Vx : Inport  Port=2
  Atan : Trigonometry  Operator=atan
  Divide : Product  Inputs=*/
  "Alfa, rad" : Outport
  wires:
  Vy/1 -> Divide/1
  Vx/1 -> Divide/2
  Divide/1 -> Atan/1
  Atan/1 -> "Alfa, rad"/1

== matlab function Model_plane9Old_vers/Динамика самолёта/Уравнения продольного движения в связанной системе координат/Subsystem/MATLAB Function ==
  data: dVx output; Vx input; Vy input; m input; Rx input; Ry input; g input; pitch input; wz input; dVy output; Iz input; M_rz input; dwz output
function [dVx,dVy,dwz] = fcn(Vx,Vy,m,Rx,Ry,g,pitch,wz,Iz,M_rz)

dVy=-wz*Vx+(Ry-m*g*cos(pitch))/m;
dVx=wz*Vy+(Rx-m*g*sin(pitch))/m;
dwz=M_rz/Iz;

== matlab function Model_plane9Old_vers/Динамика самолёта/Уравнения продольного движения в связанной системе координат/Subsystem/Рассчёт перегрузок ==
  data: Rx input; nx output; Ry input; m input; g input; ny output
function [nx, ny] = fcn(Rx, Ry, m, g)
nx=Rx/(m*g);
ny=Ry/(m*g);

== matlab function Model_plane9Old_vers/Динамика самолёта/Уравнения продольного движения в связанной системе координат/Блок расчёта пути L, высоты H, абсолютной скорости V и скорости подъёма/MATLAB Function ==
  data: Vx input; Vxg output; Vy input; pitch input; Vyg output; V output
function [Vxg,Vyg,V] = fcn(Vx,Vy,pitch)

Vxg=Vx*cos(pitch)-Vy*sin(pitch);
Vyg=Vx*sin(pitch)+Vy*cos(pitch);
V=sqrt(Vx^2+Vy^2);

== matlab function Model_plane9Old_vers/Регулятор/MATLAB Function ==
  data: Del_B input; u output; int_Del_B input; dif_Del_B input
function u = fcn(Del_B, int_Del_B, dif_Del_B)
Kp = 1.122;
K1 = 1.833;
Kd = 0.1711;

u = Kp*Del_B + K1*int_Del_B+Kd*dif_Del_B;
end

== matlab function Model_plane9Old_vers/Subsystem/MATLAB Function ==
  data: xy input; pitch output; s input
function pitch = fcn(xy,s)

pitch=atan((xy(2)-s(2))/(xy(1)-s(1)));

== matlab function Model_plane9Old_vers/Динамика самолёта/Формирование вектора состояния/MATLAB Function ==
  data: x input; s output; y input; pitch input; alfa input; V input; wz input
function s = fcn(x,y,pitch,alfa,V,wz)
s=[x,y,pitch,alfa,V,wz];

== matlab function Model_plane9Old_vers/Расчёт угла наклона руля высоты/MATLAB Function ==
  data: wz input; M_Rz input; Del_B_r output; qv input; Skr input; mz_alfa input; ba input; mz_fi input; mz_Del_B input; alfa input; alfa_t input; V input; mz_wz input; fi input; mz_alfa_t input
function Del_B_r = fcn(wz,M_Rz,qv,Skr,mz_alfa,ba,mz_fi,mz_Del_B,alfa,alfa_t,V,mz_wz,fi,mz_alfa_t)

Del_B_r=((M_Rz/(qv*Skr*ba))-((mz_wz*wz+mz_alfa_t*alfa_t)*ba/V)-mz_alfa*alfa-mz_fi*fi)/mz_Del_B;

== matlab function Model_plane9Old_vers/Динамика самолёта/Вектор внешних сил/MATLAB Function ==
  data: q input; vn output; M input; fi input
function vn = fcn(q,M,fi)

vn=[q,M,fi];

== matlab function Model_plane9Old_vers/Динамика самолёта/Блок расчёта параметров стандартной атмосферы/MATLAB Function ==
  data: ro input; a input; q output; V input; M output
function [q, M] = fcn(ro, a, V)

q=(ro*V^2)/2;
M=V/a;

== matlab function Model_plane9Old_vers/Динамика самолёта/Расчёт сил Rx, Ry по осям связанной системы координат, в которых учитывается сила тяги/Перевод аэродинамических сил из скоростной системы координат ==
  data: Ya input; X output; alfa input; Xa input; Y output
function [X,Y] = fcn(Ya,alfa,Xa)

X=Ya*sin(alfa)-Xa*cos(alfa);
Y=Ya*cos(alfa)+Xa*sin(alfa);

== matlab function Model_plane9Old_vers/Динамика самолёта/Расчёт сил Rx, Ry по осям связанной системы координат, в которых учитывается сила тяги/Проекции аэродинамических сил ==
  data: X input; Rx output; Y input; fi_p input; P input; alfa_Rud input; n_dvig input; Ry output
function [Rx, Ry] = fcn(X,Y,fi_p,P,alfa_Rud,n_dvig)

Rx=X+cos(fi_p)*(n_dvig*alfa_Rud*P);
Ry=Y+sin(fi_p)*(n_dvig*alfa_Rud*P);
